simulink model "plant"  (R2024a)
settings: Solver=VariableStepAuto  StartTime=0.0  StopTime=1000  RelTol=1e-3
settings Model: Creator=giuse  LastModifiedBy=giuse

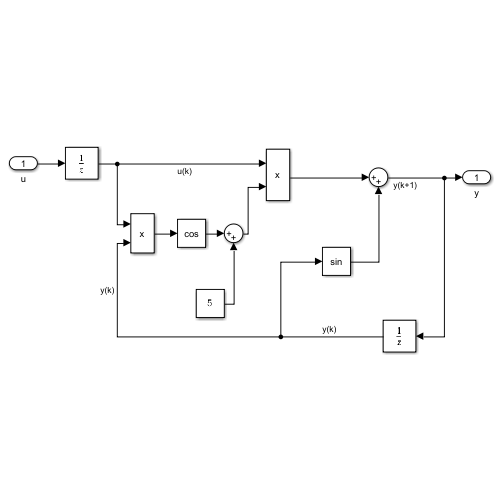
[thumbnail: Simulink's stored preview of the top-level diagram]
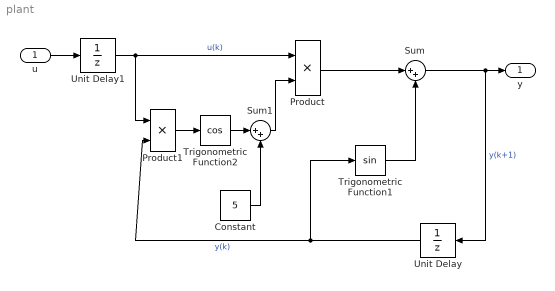
== system plant ==
  u : Inport
  Constant : Constant  Value=5
  Product : Product  RndMeth=Zero
  Product1 : Product  RndMeth=Zero
  Sum : Sum  Inputs=|++
  Sum1 : Sum  Inputs=|++
  Trigonometric Function1 : Trigonometry
  Trigonometric Function2 : Trigonometry  Operator=cos
  Unit Delay : UnitDelay
  Unit Delay1 : UnitDelay
  y : Outport
  wires:
  Trigonometric Function2/1 -> Sum1/1
  u/1 -> Unit Delay1/1
  Product/1 -> Sum/1
  Trigonometric Function1/1 -> Sum/2
  Sum/1 -> Unit Delay/1, y/1  "y(k+1)"
  Product1/1 -> Trigonometric Function2/1
  Constant/1 -> Sum1/2
  Unit Delay/1 -> Trigonometric Function1/1, Product1/2  "y(k)"
  Sum1/1 -> Product/2
  Unit Delay1/1 -> Product1/1, Product/1  "u(k)"
